simulink model "filter_bank"  (R2019b)
settings: Solver=VariableStepAuto  StartTime=0.0  StopTime=model_parameters.end  RelTol=1e-3
InitFcn:
  | [input, sampling_rate] = model_init()
undefined symbols (not defined in the file or in its folder): AXI4, Lite, model_parameters, xlfda_numerator
libraries: xbsIndex_r4 x19
settings Model: Creator=Ignazio  LastModifiedBy=Ignazio

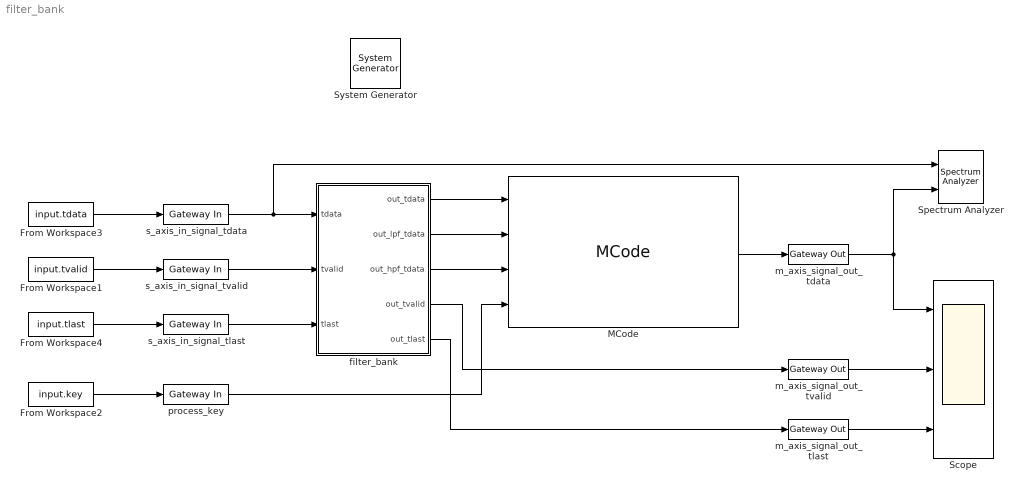
== system filter_bank ==
  " System Generator" : xbsIndex_r4/ System Generator  Tag=genX  xilinxfamily=zynquplus  part=xczu3eg  speed=-1-e  package=sbva484  synthesis_tool=Vivado  clock_wrapper=Clock Enables  directory=./generation  proj_type=Vivado  Synth_file=Vivado Synthesis Defaults  Impl_file=Vivado Implementation Defaults  testbench=off  simulink_period=1/model_parameters.sampling_rate  sysclk_period=1e9/model_parameters.sampling_rate  dcm_input_clock_period=10  incr_netlist=off  trim_vbits=Everywhere in SubSystem  dbl_ovrd=According to Block Masks  core_generation=According to Block Masks  run_coregen=off  deprecated_control=off  eval_field=0  block_type=sysgen
  From Workspace1 : FromWorkspace  VariableName=input.tvalid  SampleTime=1/model_parameters.sampling_rate  Interpolate=off  OutputAfterFinalValue=Setting to zero
  From Workspace2 : FromWorkspace  VariableName=input.key  SampleTime=1/model_parameters.sampling_rate  Interpolate=off  OutputAfterFinalValue=Setting to zero
  From Workspace3 : FromWorkspace  VariableName=input.tdata  SampleTime=1/model_parameters.sampling_rate  Interpolate=off  OutputAfterFinalValue=Setting to zero
  From Workspace4 : FromWorkspace  VariableName=input.tlast  SampleTime=1/model_parameters.sampling_rate  Interpolate=off  OutputAfterFinalValue=Setting to zero
  MCode : xbsIndex_r4/MCode  mfname=switch_output  explicit_period=off  period=1  inputsTable={'boundInpExpr'=>['','','',''],'inputs'=>['inputArg0','inputArg1','inputArg2','selector']}  outputsTable={'outputs'=>['output_signal'],'suppressOut'=>['off']}  enable_stdout=off  enable_debug=off  suppress_output=on  defparams={}  hide_port_list={}  dbl_ovrd=off  block_type=mcode
  Scope : Scope  NumInputPorts=3
  Spectrum Analyzer : SpectrumAnalyzer  NumInputPorts=2
  filter_bank : Subsystem
  m_axis_signal_out_tdata : xbsIndex_r4/Gateway Out  inherit_from_input=off  hdl_port=on  rows=1  columns=1  UseAsDAC=off  DACChannel='1'  interface=None  automatic_assignment=on  address_offset=hex2dec('00')  intf_name=''  intf_description=''  timing_constraint=None  locs_specified=off  LOCs={}  io_standard={}  block_type=gatewayout
  m_axis_signal_out_tlast : xbsIndex_r4/Gateway Out  inherit_from_input=off  hdl_port=on  rows=1  columns=1  UseAsDAC=off  DACChannel='1'  interface=None  automatic_assignment=on  address_offset=hex2dec('00')  intf_name=''  intf_description=''  timing_constraint=None  locs_specified=off  LOCs={}  io_standard={}  block_type=gatewayout
  m_axis_signal_out_tvalid : xbsIndex_r4/Gateway Out  inherit_from_input=off  hdl_port=on  rows=1  columns=1  UseAsDAC=off  DACChannel='1'  interface=None  automatic_assignment=on  address_offset=hex2dec('00')  intf_name=''  intf_description=''  timing_constraint=None  locs_specified=off  LOCs={}  io_standard={}  block_type=gatewayout
  process_key : xbsIndex_r4/Gateway In  gui_display_data_type=Fixed-point  arith_type=Unsigned  n_bits=8  bin_pt=0  preci_type=Single  exp_width=8  frac_width=24  rows=1  columns=1  quantization="Round  (unbiased: +/- Inf)"  overflow=Saturate  period=1/model_parameters.sampling_rate  UseAsADC=off  ADCChannel='1'  interface=AXI4-Lite  automatic_assignment=on  address_offset=hex2dec('00')  intf_name=''  intf_description=''  default_value=0  timing_constraint=None  locs_specified=off  LOCs={}  io_standard={}  inherit_from_input=off  hdl_port=on  dbl_ovrd=off  block_type=gatewayin
  s_axis_in_signal_tdata : xbsIndex_r4/Gateway In  gui_display_data_type=Fixed-point  arith_type="Signed  (2's comp)"  n_bits=16  bin_pt=14  preci_type=Single  exp_width=8  frac_width=24  rows=1  columns=1  quantization="Round  (unbiased: +/- Inf)"  overflow=Saturate  period=1/model_parameters.sampling_rate  UseAsADC=off  ADCChannel='1'  interface=None  automatic_assignment=on  address_offset=hex2dec('00')  intf_name=''  intf_description=''  default_value=0  timing_constraint=None  locs_specified=off  LOCs={}  io_standard={}  inherit_from_input=off  hdl_port=on  dbl_ovrd=off  block_type=gatewayin
  s_axis_in_signal_tlast : xbsIndex_r4/Gateway In  gui_display_data_type=Boolean  arith_type=Boolean  n_bits=16  bin_pt=14  preci_type=Single  exp_width=8  frac_width=24  rows=1  columns=1  quantization="Round  (unbiased: +/- Inf)"  overflow=Saturate  period=1/model_parameters.sampling_rate  UseAsADC=off  ADCChannel='1'  interface=None  automatic_assignment=on  address_offset=hex2dec('00')  intf_name=''  intf_description=''  default_value=0  timing_constraint=None  locs_specified=off  LOCs={}  io_standard={}  inherit_from_input=off  hdl_port=on  dbl_ovrd=off  block_type=gatewayin
  s_axis_in_signal_tvalid : xbsIndex_r4/Gateway In  gui_display_data_type=Boolean  arith_type=Boolean  n_bits=16  bin_pt=14  preci_type=Single  exp_width=8  frac_width=24  rows=1  columns=1  quantization="Round  (unbiased: +/- Inf)"  overflow=Saturate  period=1/model_parameters.sampling_rate  UseAsADC=off  ADCChannel='1'  interface=None  automatic_assignment=on  address_offset=hex2dec('00')  intf_name=''  intf_description=''  default_value=0  timing_constraint=None  locs_specified=off  LOCs={}  io_standard={}  inherit_from_input=off  hdl_port=on  dbl_ovrd=off  block_type=gatewayin
  wires:
  process_key/1 -> MCode/4
  MCode/1 -> m_axis_signal_out_tdata/1
  From Workspace3/1 -> s_axis_in_signal_tdata/1
  s_axis_in_signal_tdata/1 -> Spectrum Analyzer/1, filter_bank/1(tdata)
  s_axis_in_signal_tvalid/1 -> filter_bank/2(tvalid)
  s_axis_in_signal_tlast/1 -> filter_bank/3(tlast)
  filter_bank/1(out_tdata) -> MCode/1
  filter_bank/2(out_lpf_tdata) -> MCode/2
  filter_bank/3(out_hpf_tdata) -> MCode/3
  filter_bank/4(out_tvalid) -> m_axis_signal_out_tvalid/1
  filter_bank/5(out_tlast) -> m_axis_signal_out_tlast/1
  From Workspace1/1 -> s_axis_in_signal_tvalid/1
  From Workspace4/1 -> s_axis_in_signal_tlast/1
  From Workspace2/1 -> process_key/1
  m_axis_signal_out_tdata/1 -> Scope/1, Spectrum Analyzer/2
  m_axis_signal_out_tvalid/1 -> Scope/2
  m_axis_signal_out_tlast/1 -> Scope/3

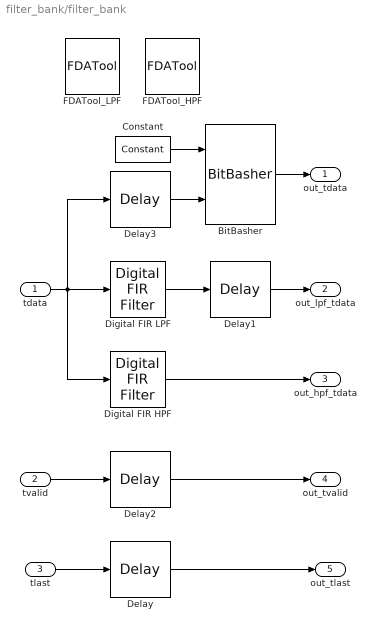
== system filter_bank/filter_bank ==
  tdata : Inport
  tvalid : Inport  Port=2
  tlast : Inport  Port=3
  BitBasher : xbsIndex_r4/BitBasher  bitexpr=a={b,c}  display_expr=off  sr_1=a  arith_type1="Signed  (2's comp)"  bin_pt1=28  sr_2=2  arith_type2=Unsigned  bin_pt2=0  sr_3=3  arith_type3=Unsigned  bin_pt3=0  sr_4=4  arith_type4=Unsigned  bin_pt4=0  dbl_ovrd=off  block_type=bitbasher
  Constant : xbsIndex_r4/Constant  const=0  gui_display_data_type=Fixed-point  arith_type=Unsigned  n_bits=16  bin_pt=0  preci_type=Single  exp_width=8  frac_width=24  explicit_period=off  period=1  equ=P=C  opselect=C  inp2=PCIN>>17  opr=+  inp1=P  carry=CIN  dbl_ovrd=off  block_type=constant
  Delay : xbsIndex_r4/Delay  rst=off  infoeditControl=Selection of Reset will increase slice count due to use of real FFs and instead of SRLs  en=off  latency=28  reg_retiming=off  dbl_ovrd=off  block_type=delay
  Delay1 : xbsIndex_r4/Delay  rst=off  infoeditControl=Selection of Reset will increase slice count due to use of real FFs and instead of SRLs  en=off  latency=3  reg_retiming=off  dbl_ovrd=off  block_type=delay
  Delay2 : xbsIndex_r4/Delay  rst=off  infoeditControl=Selection of Reset will increase slice count due to use of real FFs and instead of SRLs  en=off  latency=28  reg_retiming=off  dbl_ovrd=off  block_type=delay
  Delay3 : xbsIndex_r4/Delay  rst=off  infoeditControl=Selection of Reset will increase slice count due to use of real FFs and instead of SRLs  en=off  latency=28  reg_retiming=off  dbl_ovrd=off  block_type=delay
  Digital FIR HPF : xbsIndex_r4/Digital FIR Filter  coeff_source=off  coefficientvector=xlfda_numerator('FDATool_HPF')  coeff_calulate=off  coefficient_width=16  coefficient_fractional_bits=14  interpolation_filter_rate=1  decimation_filter_rate=1  fda_coefficientvector=[-0.00148645269921017 0.00526328031957434 -0.00649180404223257 -0.000501828025987646 0.00893346166427297 -0.00586983903830583 -0.00314558643105247 0.000197099423364437 0.0091114790175841 -0.00340242484917138 -0.00787133312869585 -0.0008250206272161 0.0131228466370689 0.000787674406030639 -0.0142446546069574 -0.00605394764881058 0.0190689858656729 0.0102041827169008 -0.0213081469368879 -0.0194456971410297 0.0254244439845981 0.031358565343375 -0.0275391485134136 -0.0535218772011121 0.0303319224270644 0.0993363133610281 -0.0312217954042448 -0.316331884141437 0.532181223103044 -0.316331884141437 -0.0312217954042448 0.0993363133610281 0.0303319224270644 -0.0535218772011121 -0.0275391485134136 0.031358565343375 0.0254244439845981 -0.0194456971410297 -0.0213081469368879 0.0102041827169008 0.0190689858656729 -0.00605394764881058 -0.0142446546069574 0.000787674406030639 0.0131228466370689 -0.0008250206272161 -0.00787133312869585 -0.00340242484917138 0.0091114790175841 0.000197099423364437 -0.00314558643105247 -0.00586983903830583 0.00893346166427297 -0.000501828025987646 -0.00649180404223257 0.00526328031957434 -0.00148645269921017]  simulation_type=fast_sim  simulation_model=sysgen:fir_macro  block_type=fir_macro
  Digital FIR LPF : xbsIndex_r4/Digital FIR Filter  coeff_source=off  coefficientvector=xlfda_numerator('FDATool_LPF')  coeff_calulate=off  coefficient_width=16  coefficient_fractional_bits=14  interpolation_filter_rate=1  decimation_filter_rate=1  fda_coefficientvector=[-0.000922175232821972 -0.00273958133317832 -0.00255036555988357 0.00355621457714135 0.0135493675450094 0.0173158167843651 0.00770838306531653 -0.00649307059052154 -0.00768045146622222 0.00608565944583592 0.0138781398261134 0.000396827974269109 -0.016872825891288 -0.00891939395727656 0.0174119503029707 0.0207545927500639 -0.0122604496044705 -0.0342350688782289 -0.00106574117850845 0.0477779205992946 0.0273960894331456 -0.0593497624727359 -0.0823259890492311 0.0671522204513427 0.310023479333045 0.430087585178213 0.310023479333045 0.0671522204513427 -0.0823259890492311 -0.0593497624727359 0.0273960894331456 0.0477779205992946 -0.00106574117850845 -0.0342350688782289 -0.0122604496044705 0.0207545927500639 0.0174119503029707 -0.00891939395727656 -0.016872825891288 0.000396827974269109 0.0138781398261134 0.00608565944583592 -0.00768045146622222 -0.00649307059052154 0.00770838306531653 0.0173158167843651 0.0135493675450094 0.00355621457714135 -0.00255036555988357 -0.00273958133317832 -0.000922175232821972]  simulation_type=fast_sim  simulation_model=sysgen:fir_macro  block_type=fir_macro
  FDATool_HPF : xbsIndex_r4/FDATool  block_type=fdatool
      settings: infoedit=FDATool
  FDATool_LPF : xbsIndex_r4/FDATool  block_type=fdatool
      settings: infoedit=FDATool
  out_tdata : Outport
  out_lpf_tdata : Outport  Port=2
  out_hpf_tdata : Outport  Port=3
  out_tvalid : Outport  Port=4
  out_tlast : Outport  Port=5
  wires:
  Digital FIR HPF/1 -> out_hpf_tdata/1
  Digital FIR LPF/1 -> Delay1/1
  tdata/1 -> Digital FIR HPF/1, Delay3/1, Digital FIR LPF/1
  tlast/1 -> Delay/1
  Delay1/1 -> out_lpf_tdata/1
  Delay2/1 -> out_tvalid/1
  Delay/1 -> out_tlast/1
  tvalid/1 -> Delay2/1
  Delay3/1 -> BitBasher/2
  BitBasher/1 -> out_tdata/1
  Constant/1 -> BitBasher/1
